simulink model "Kalman_State_Estimation"  (R2016b)
settings: Solver=VariableStepAuto  StartTime=0.0  StopTime=30  RelTol=1e-3
values from neighbouring files (symbols this model uses):
  A = [1 1 0;0 1 1;0 0 1]    [kalman_script.m]
  theta = 70    [kalman_script.m]
undefined symbols (not defined in the file or in its folder): Discrete, Time
libraries: ctrlSharedLib x1
settings Model: Creator=karanverma  LastModifiedBy=karanverma

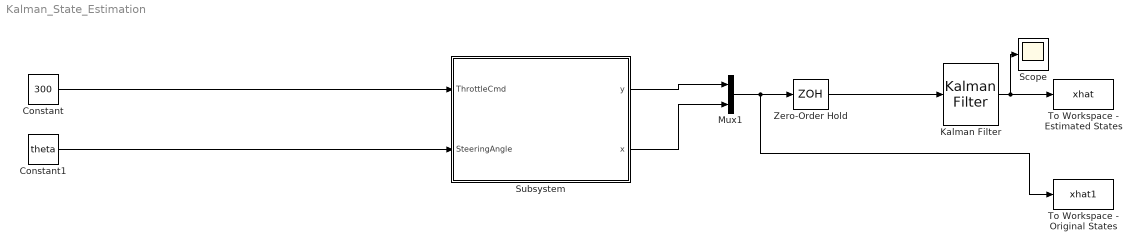
== system Kalman_State_Estimation ==
  Constant : Constant  Value=300
  Constant1 : Constant  Value=theta
  Kalman Filter : ctrlSharedLib/Kalman Filter  TimeDomain=Discrete-Time  UseCurrentEstimator=on  ModelSource=Individual A, B, C, D matrices  ModelSourceVariable=sys  A=A  B=1  C=[1 0 0;0 0 1]  D=0  NumberOfStates=1  NumberOfInputs=1  NumberOfOutputs=1  InitialEstimateSource=Dialog  X0=0  P0=10  UseK=off  UseGH=off  NumberOfProcessNoiseInputs=1  G=1  TimeInvariantG=on  H=0  TimeInvariantH=on  Q=0.05  TimeInvariantQ=on  R=10  TimeInvariantR=on  N=0  TimeInvariantN=on  AddInputPort=off  AddEnablePort=off  OutputEstimatedY=off  OutputP=off  Ts=-1
  Mux1 : Mux  Inputs=2
  Scope : Scope
  Subsystem : Subsystem
  To Workspace - Estimated States : ToWorkspace  VariableName=xhat  SampleTime=-1
      settings: Save2DSignal=2-D array (concatenate along first dimension)
  "To Workspace - Original States " : ToWorkspace  VariableName=xhat1  SampleTime=-1
      settings: Save2DSignal=2-D array (concatenate along first dimension)
  Zero-Order Hold : ZeroOrderHold
  wires:
  Constant/1 -> Subsystem/1(ThrottleCmd)
  Constant1/1 -> Subsystem/2(SteeringAngle)
  Subsystem/2(x) -> Mux1/2
  Subsystem/1(y) -> Mux1/1
  Mux1/1 -> "To Workspace - Original States "/1, Zero-Order Hold/1
  Zero-Order Hold/1 -> Kalman Filter/1
  Kalman Filter/1 -> Scope/1, To Workspace - Estimated States/1

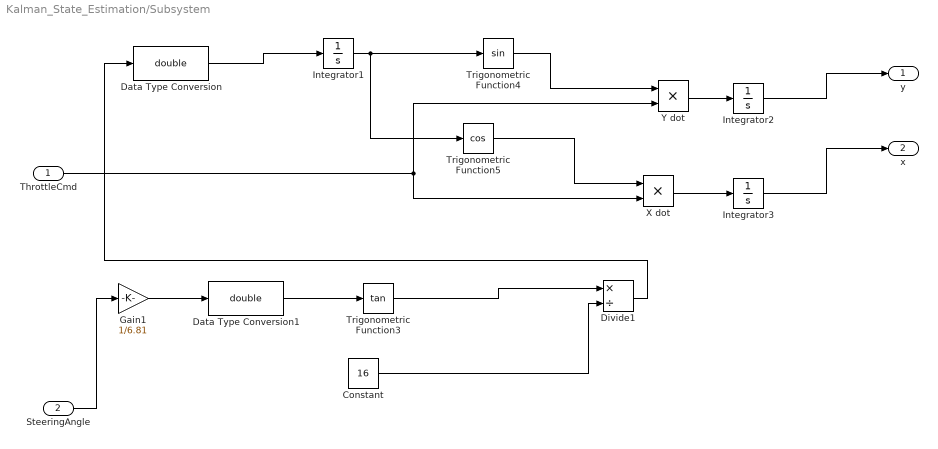
== system Kalman_State_Estimation/Subsystem ==
  ThrottleCmd : Inport
  SteeringAngle : Inport  Port=2
  Constant : Constant  Value=16
  Data Type Conversion : DataTypeConversion  OutDataTypeStr=double
  Data Type Conversion1 : DataTypeConversion  OutDataTypeStr=double
  Divide1 : Product  Inputs=*/
  Gain1 : Gain  Gain=1/6.81
  Integrator1 : Integrator
  Integrator2 : Integrator
  Integrator3 : Integrator
  Trigonometric Function3 : Trigonometry  Operator=tan  OutputSignalType=real
  Trigonometric Function4 : Trigonometry
  Trigonometric Function5 : Trigonometry  Operator=cos
  "X dot " : Product
  "Y dot " : Product
  y : Outport
  x : Outport  Port=2
  wires:
  Gain1/1 -> Data Type Conversion1/1
  Integrator1/1 -> Trigonometric Function5/1, Trigonometric Function4/1
  ThrottleCmd/1 -> "X dot "/2, "Y dot "/2
  Trigonometric Function5/1 -> "X dot "/1
  Trigonometric Function4/1 -> "Y dot "/1
  "X dot "/1 -> Integrator3/1
  "Y dot "/1 -> Integrator2/1
  Data Type Conversion/1 -> Integrator1/1
  Integrator2/1 -> y/1
  Integrator3/1 -> x/1
  SteeringAngle/1 -> Gain1/1
  Data Type Conversion1/1 -> Trigonometric Function3/1
  Trigonometric Function3/1 -> Divide1/1
  Constant/1 -> Divide1/2
  Divide1/1 -> Data Type Conversion/1
